simulink model "SVPWM"  (R2023b)
settings: Solver=FixedStepAuto  StartTime=0.0  StopTime=10.0  FixedStep=1e-4  RelTol=1e-3
undefined symbols (not defined in the file): curr_d_ki, curr_d_kp, curr_q_ki, curr_q_kp, CurrKi, CurrKp, Pn, Udc
libraries: slpidlib x4, mcbplantlib x1, autolibpmsmexterior x1
settings Model: DataDictionary=FOC.sldd  Creator=18575  LastModifiedBy=18575
settings OptimizationCC: DefaultParameterBehavior=Inlined  UseDivisionForNetSlopeComputation=on  GainParamInheritBuiltInType=on  UseFloatMulNetSlope=on  InlineInvariantSignals=on  PassReuseOutputArgsAs=Individual arguments  ZeroExternalMemoryAtStartup=off  ZeroInternalMemoryAtStartup=off  NoFixptDivByZeroProtection=on  EfficientFloat2IntCast=on  LifeSpan=1  OptimizeBlockOrder=speed  DifferentSizesBufferReuse=on  EfficientTunableParamExpr=on
settings DebuggingCC: ParameterTunabilityLossMsg=error
settings HardwareCC: ProdBitPerPointer=32  ProdBitPerSizeT=32  ProdBitPerPtrDiffT=32  ProdLargestAtomicInteger=Long  ProdLargestAtomicFloat=Double  ProdWordSize=32  ProdLongLongMode=on  ProdHWDeviceType=ARM Compatible->ARM Cortex-M
settings SFSimCC: MATLABDynamicMemAlloc=off
settings RTWCC: Description=Embedded Coder  SystemTargetFile=ert.tlc  TemplateMakefile=ert_default_tmf  GenerateReport=on  LaunchReport=on
settings CodeAppCC: ForceParamTrailComments=on  IgnoreCustomStorageClasses=off  OperatorAnnotations=on  SimulinkDataObjDesc=on  SFDataObjDesc=on  CustomSymbolStrGlobalVar=rt$N$M  CustomSymbolStrType=$N$M  CustomSymbolStrFcn=$N$M$F  CustomSymbolStrMacro=$N$M  InsertBlockDesc=on
settings ERTTargetCC: TargetLangStandard=C99 (ISO)  CodeReplacementLibrary=ARM Cortex-M  GenerateSampleERTMain=on  IncludeMdlTerminateFcn=off  CombineSignalStateStructs=on  SuppressErrorStatus=on  SupportAbsoluteTime=off  SupportNonFinite=off  SupportComplex=off  InlinedParameterPlacement=NonHierarchical  ERTCustomFileTemplate=example_file_process.tlc  ERTFilePackagingFormat=CompactWithDataFile

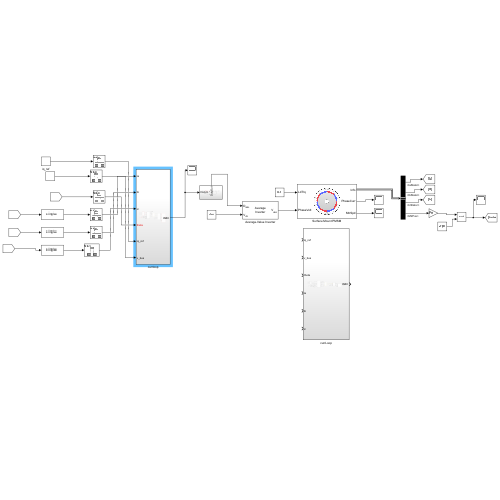
[thumbnail: Simulink's stored preview of the top-level diagram]
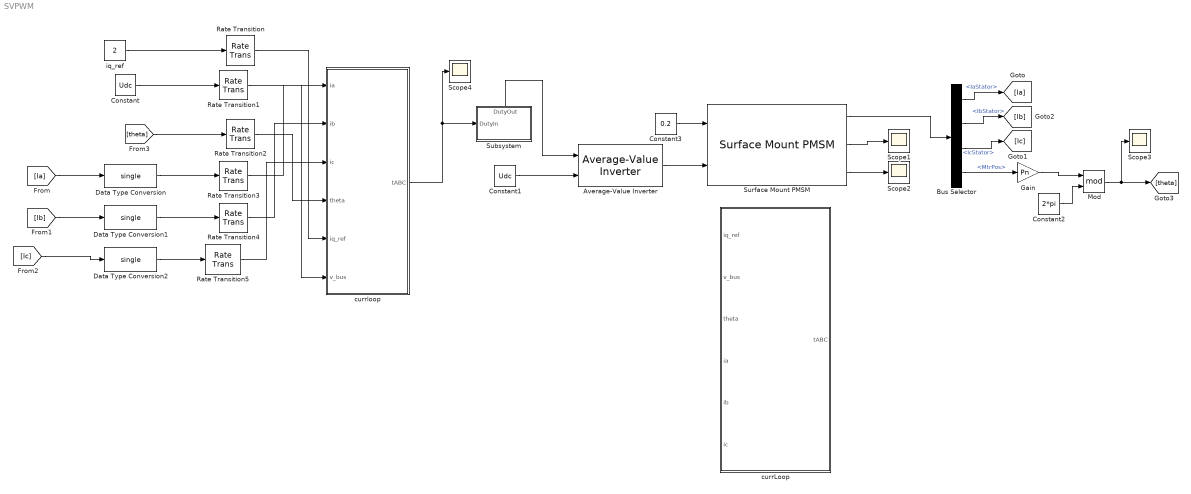
== system SVPWM ==
  Average-Value Inverter : mcbplantlib/Average-Value Inverter
      settings: LibrarySourceBlock=mcblib/Electrical Systems/Inverters/Average-Value Inverter
  Bus Selector : BusSelector  OutputSignals=IaStator,IbStator,IcStator,MtrPos
  Constant : Constant  Value=Udc
  Constant1 : Constant  Value=Udc
  Constant2 : Constant  Value=2*pi
  Constant3 : Constant  Value=0.2
  Data Type Conversion : DataTypeConversion  OutDataTypeStr=single  SaturateOnIntegerOverflow=off  RndMeth=Floor
  Data Type Conversion1 : DataTypeConversion  OutDataTypeStr=single  SaturateOnIntegerOverflow=off  RndMeth=Floor
  Data Type Conversion2 : DataTypeConversion  OutDataTypeStr=single  SaturateOnIntegerOverflow=off  RndMeth=Floor
  Gain : Gain  Gain=Pn
  Mod : Math  Operator=mod
  Rate Transition{,1..5} (6 alike) : RateTransition
  Scope{1..4} (4 alike) : Scope
  Subsystem : Subsystem
      settings: PortSchema="{\"entries\":[{\"content\":{\"sides\":[{\"content\":{\"connectorIds\":[\"In1\"]},\"type\":\"ConnectorPlacement.EquallySpacedRectSide\",\"uuid\":\"8ccc51de-fa2a-4900-80a3-4cdf9aa76f01\"},{\"content\":{\"side\":\"RIGHT\"},\"type\":\"ConnectorPlacement.EquallySpacedRectSide\",\"uuid\":\"32c06e0d-3f1d-4948-af96-e310e54308a0\"},{\"content\":{\"connectorIds\":[\"Out1\"],\"side\":\"TOP\"},\"type\":\"ConnectorPlacement.EquallySpacedRectSide\",\"uuid\":\"a9066067-2c54-42a8-b4d7-fb86ac71b860\"}]},\"type\":\"ConnectorPlacement.EquallySpacedConnector\",\"uuid\":\"e4576975-acad-4e16-822f-2c2e7f23d7a7\"}],\"packageUris\":[\"http://schema.mathworks.com/mf0/Connector/R2020b\"],\"version\":\"1.0\"}"
  Surface Mount PMSM : autolibpmsmexterior/Surface Mount PMSM  port_config=Torque  sim_type=Discrete  Ts=1e-4  FilePath=E:\Sandbox\Bauto\Work\surfacepmsm_motordata.m  P=Pn  Rs=Rs  Ldq_=L  KConstText=Permanent flux linkage constant (lambda_pm):  lambda_pm=flux  Ke=159.9771  Kt=1.323  mechanical=[75e-6, 8e-5, 0]  idq0=[0 0]  theta_init=0  omega_init=0  KConst=flux  lambda_pm_calc=flux  RefBlkName='autolibpmsmexterior/Surface Mount PMSM'  aMode=1  Ldq="[0.0003752   0.0003752]"
      settings: LibrarySourceBlock=autolibemachines/Surface Mount PMSM
  currLoop : Subsystem
  currloop : Subsystem
  iq_ref : Constant  Value=2  OutDataTypeStr=single
  wires:
  Average-Value Inverter/1 -> Surface Mount PMSM/2
  Surface Mount PMSM/3 -> Scope2/1
  Surface Mount PMSM/2 -> Scope1/1
  Surface Mount PMSM/1 -> Bus Selector/1
  iq_ref/1 -> Rate Transition/1
  Constant/1 -> Rate Transition1/1
  [theta] -> Rate Transition2/1
  currloop/1(tABC) -> Scope4/1, Subsystem/1(DutyIn)
  Subsystem/1(DutyOut) -> Average-Value Inverter/1
  [Ia] -> Data Type Conversion/1
  [Ic] -> Data Type Conversion2/1
  [Ib] -> Data Type Conversion1/1
  Data Type Conversion/1 -> Rate Transition3/1
  Data Type Conversion1/1 -> Rate Transition4/1
  Data Type Conversion2/1 -> Rate Transition5/1
  Rate Transition/1 -> currloop/5(iq_ref)
  Rate Transition1/1 -> currloop/6(v_bus)
  Rate Transition2/1 -> currloop/4(theta)
  Rate Transition3/1 -> currloop/1(ia)
  Rate Transition4/1 -> currloop/2(ib)
  Rate Transition5/1 -> currloop/3(ic)
  Bus Selector/1 -> [Ia]  "<IaStator>"
  Bus Selector/2 -> [Ib]  "<IbStator>"
  Bus Selector/3 -> [Ic]  "<IcStator>"
  Bus Selector/4 -> Gain/1  "<MtrPos>"
  Constant1/1 -> Average-Value Inverter/2
  Gain/1 -> Mod/1
  Constant2/1 -> Mod/2
  Mod/1 -> Scope3/1, [theta]
  Constant3/1 -> Surface Mount PMSM/1

== system SVPWM/Subsystem ==
  DutyIn : Inport
  Constant : Constant  Value=0.5  SampleTime=-1
  Gain : Gain  Gain=1/8000  ParamDataTypeStr=single
  Gain1 : Gain  Gain=-1
  Sum : Sum  Inputs=|+-
  Sum1 : Sum  Inputs=|++
  DutyOut : Outport
  wires:
  Sum/1 -> Gain1/1
  Constant/1 -> Sum1/2, Sum/2
  DutyIn/1 -> Gain/1
  Gain1/1 -> Sum1/1
  Sum1/1 -> DutyOut/1
  Gain/1 -> Sum/1

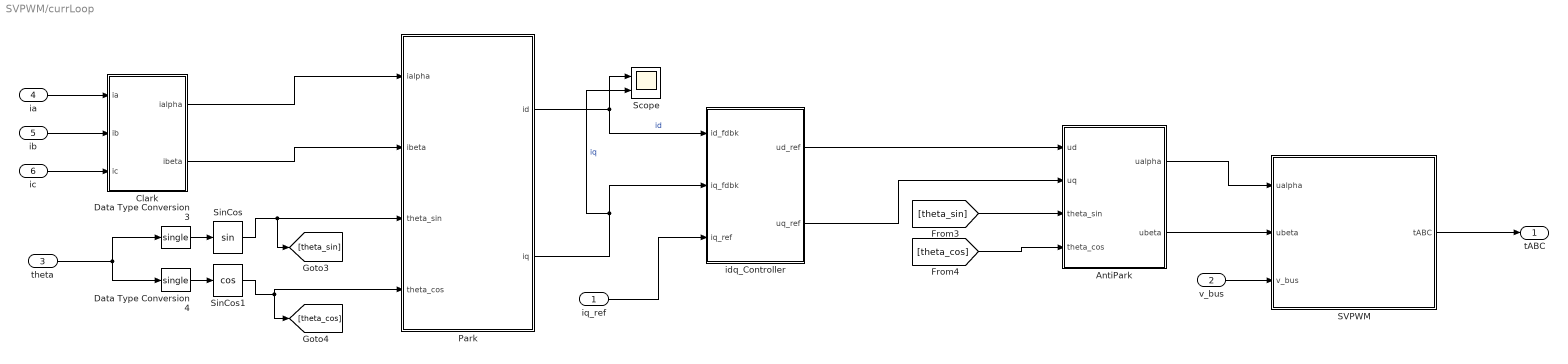
== system SVPWM/currLoop ==
  iq_ref : Inport
  v_bus : Inport  Port=2
  theta : Inport  Port=3
  ia : Inport  Port=4
  ib : Inport  Port=5
  ic : Inport  Port=6
  AntiPark : Subsystem
  Clark : Subsystem
  Data Type Conversion3 : DataTypeConversion  OutDataTypeStr=single  SaturateOnIntegerOverflow=off  RndMeth=Floor
  Data Type Conversion4 : DataTypeConversion  OutDataTypeStr=single  SaturateOnIntegerOverflow=off  RndMeth=Floor
  Park : Subsystem
  SVPWM : Subsystem
  Scope : Scope  NumInputPorts=2
  SinCos : Trigonometry
  SinCos1 : Trigonometry  Operator=cos
  idq_Controller : Subsystem
  tABC : Outport
  wires:
  v_bus/1 -> SVPWM/3(v_bus)
  Park/1(id) -> idq_Controller/1(id_fdbk), Scope/1  "id"
  SVPWM/1(tABC) -> tABC/1
  [theta_sin] -> AntiPark/3(theta_sin)
  SinCos/1 -> Park/3(theta_sin), [theta_sin]
  theta/1 -> Data Type Conversion4/1, Data Type Conversion3/1
  [theta_cos] -> AntiPark/4(theta_cos)
  idq_Controller/1(ud_ref) -> AntiPark/1(ud)
  SinCos1/1 -> Park/4(theta_cos), [theta_cos]
  AntiPark/2(ubeta) -> SVPWM/2(ubeta)
  AntiPark/1(ualpha) -> SVPWM/1(ualpha)
  idq_Controller/2(uq_ref) -> AntiPark/2(uq)
  Park/2(iq) -> idq_Controller/2(iq_fdbk), Scope/2  "iq"
  Clark/2(ibeta) -> Park/2(ibeta)
  iq_ref/1 -> idq_Controller/3(iq_ref)
  Clark/1(ialpha) -> Park/1(ialpha)
  Data Type Conversion4/1 -> SinCos1/1
  Data Type Conversion3/1 -> SinCos/1
  ia/1 -> Clark/1(ia)
  ib/1 -> Clark/2(ib)
  ic/1 -> Clark/3(ic)

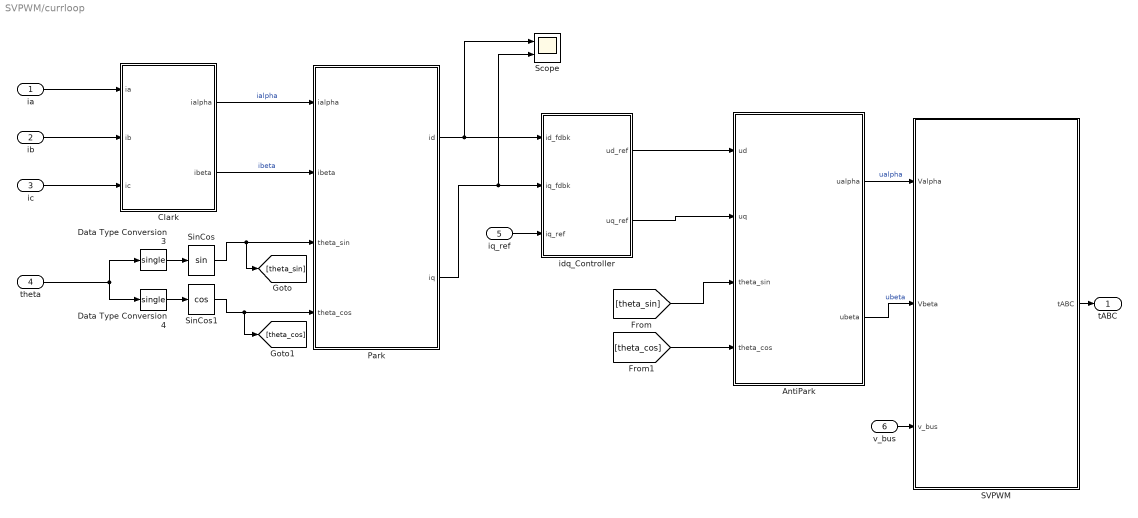
== system SVPWM/currloop ==
  ia : Inport
  ib : Inport  Port=2
  ic : Inport  Port=3
  theta : Inport  Port=4
  iq_ref : Inport  Port=5
  v_bus : Inport  Port=6
  AntiPark : Subsystem
  Clark : Subsystem
  Data Type Conversion3 : DataTypeConversion  OutDataTypeStr=single  SaturateOnIntegerOverflow=off  RndMeth=Floor
  Data Type Conversion4 : DataTypeConversion  OutDataTypeStr=single  SaturateOnIntegerOverflow=off  RndMeth=Floor
  Park : Subsystem
  SVPWM : Subsystem  TreatAsAtomicUnit=on
  Scope : Scope  NumInputPorts=2
  SinCos : Trigonometry
  SinCos1 : Trigonometry  Operator=cos
  idq_Controller : Subsystem
  tABC : Outport
  wires:
  Data Type Conversion4/1 -> SinCos1/1
  Data Type Conversion3/1 -> SinCos/1
  AntiPark/2(ubeta) -> SVPWM/2(Vbeta)  "ubeta"
  AntiPark/1(ualpha) -> SVPWM/1(Valpha)  "ualpha"
  [theta_cos] -> AntiPark/4(theta_cos)
  [theta_sin] -> AntiPark/3(theta_sin)
  SinCos/1 -> Park/3(theta_sin), [theta_sin]
  theta/1 -> Data Type Conversion3/1, Data Type Conversion4/1
  SinCos1/1 -> Park/4(theta_cos), [theta_cos]
  v_bus/1 -> SVPWM/3(v_bus)
  SVPWM/1(tABC) -> tABC/1
  ib/1 -> Clark/2(ib)
  ia/1 -> Clark/1(ia)
  ic/1 -> Clark/3(ic)
  Clark/1(ialpha) -> Park/1(ialpha)  "ialpha"
  Clark/2(ibeta) -> Park/2(ibeta)  "ibeta"
  idq_Controller/1(ud_ref) -> AntiPark/1(ud)
  idq_Controller/2(uq_ref) -> AntiPark/2(uq)
  Park/1(id) -> Scope/1, idq_Controller/1(id_fdbk)
  Park/2(iq) -> Scope/2, idq_Controller/2(iq_fdbk)
  iq_ref/1 -> idq_Controller/3(iq_ref)

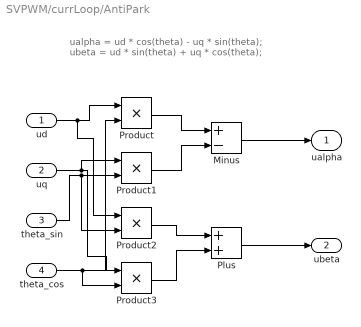
== system SVPWM/currLoop/AntiPark ==
  note: ualpha = ud * cos(theta) - uq * sin(theta);
      | ubeta = ud * sin(theta) + uq * cos(theta);
  ud : Inport
  uq : Inport  Port=2
  theta_sin : Inport  Port=3
  theta_cos : Inport  Port=4
  Minus : Sum  Inputs=+-
  Plus : Sum
  Product{,1..3} (4 alike) : Product
  ualpha : Outport
  ubeta : Outport  Port=2
  wires:
  ud/1 -> Product2/1, Product/1
  theta_cos/1 -> Product3/2, Product/2
  Product/1 -> Minus/1
  uq/1 -> Product3/1, Product1/1
  theta_sin/1 -> Product2/2, Product1/2
  Product1/1 -> Minus/2
  Minus/1 -> ualpha/1
  Product2/1 -> Plus/1
  Product3/1 -> Plus/2
  Plus/1 -> ubeta/1

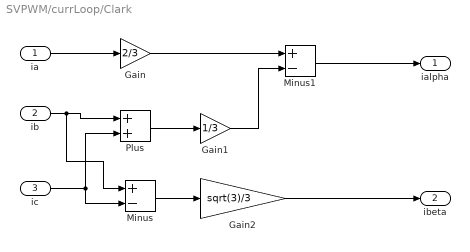
== system SVPWM/currLoop/Clark ==
  ia : Inport  OutDataTypeStr=single
  ib : Inport  Port=2  OutDataTypeStr=single
  ic : Inport  Port=3  OutDataTypeStr=single
  Gain : Gain  Gain=2/3
  Gain1 : Gain  Gain=1/3
  Gain2 : Gain  Gain=sqrt(3)/3
  Minus : Sum  Inputs=+-
  Minus1 : Sum  Inputs=+-
  Plus : Sum
  ialpha : Outport
  ibeta : Outport  Port=2
  wires:
  Gain/1 -> Minus1/1
  Plus/1 -> Gain1/1
  ic/1 -> Minus/2, Plus/2
  Gain1/1 -> Minus1/2
  Gain2/1 -> ibeta/1
  Minus1/1 -> ialpha/1
  ia/1 -> Gain/1
  Minus/1 -> Gain2/1
  ib/1 -> Minus/1, Plus/1

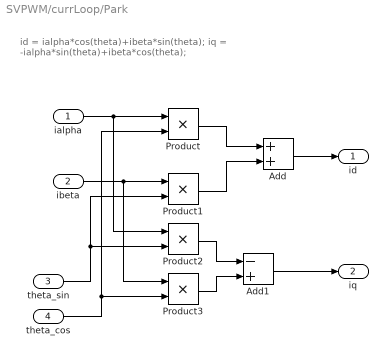
== system SVPWM/currLoop/Park ==
  note: id = ialpha*cos(theta)+ibeta*sin(theta);
      | iq = -ialpha*sin(theta)+ibeta*cos(theta);
  ialpha : Inport  OutDataTypeStr=single
  ibeta : Inport  Port=2  OutDataTypeStr=single
  theta_sin : Inport  Port=3  OutDataTypeStr=single
  theta_cos : Inport  Port=4  OutDataTypeStr=single
  Add : Sum  OutDataTypeStr=single  AccumDataTypeStr=single
  Add1 : Sum  Inputs=-+  OutDataTypeStr=single  AccumDataTypeStr=single
  Product{,1..3} (4 alike) : Product  OutDataTypeStr=single
  id : Outport  OutDataTypeStr=single
  iq : Outport  Port=2  OutDataTypeStr=single
  wires:
  theta_sin/1 -> Product2/2, Product1/2
  Product/1 -> Add/1
  Product2/1 -> Add1/1
  ialpha/1 -> Product2/1, Product/1
  Product3/1 -> Add1/2
  Add/1 -> id/1
  Add1/1 -> iq/1
  Product1/1 -> Add/2
  ibeta/1 -> Product3/1, Product1/1
  theta_cos/1 -> Product3/2, Product/2

== system SVPWM/currLoop/SVPWM ==
  ualpha : Inport
  ubeta : Inport  Port=2
  v_bus : Inport  Port=3
  AntiClark : Subsystem
  Divide : Product  Inputs=*/
  Mux : Mux  Inputs=3
  PWM_halfPeriod : Gain  Gain=8000
  Sum : Sum  Inputs=++|
  center : Subsystem
  tABC : Outport
  wires:
  AntiClark/1(Ua) -> Mux/1
  AntiClark/2(Ub) -> Mux/2
  AntiClark/3(Uc) -> Mux/3
  Mux/1 -> Sum/2, center/1(Uabc)
  center/1(Ucenter) -> Sum/1
  v_bus/1 -> Divide/2, center/2(v_bus)
  ualpha/1 -> AntiClark/1(ualpha)
  ubeta/1 -> AntiClark/2(ubeta)
  Sum/1 -> Divide/1
  Divide/1 -> PWM_halfPeriod/1
  PWM_halfPeriod/1 -> tABC/1

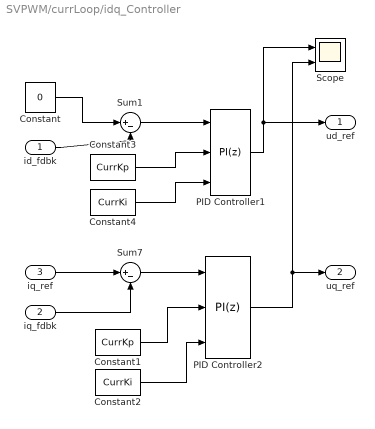
== system SVPWM/currLoop/idq_Controller ==
  id_fdbk : Inport  OutDataTypeStr=single
  iq_fdbk : Inport  Port=2  OutDataTypeStr=single
  iq_ref : Inport  Port=3  OutDataTypeStr=single
  Constant : Constant  Value=0  OutDataTypeStr=single
  Constant1 : Constant  Value=CurrKp  OutDataTypeStr=single
  Constant2 : Constant  Value=CurrKi  OutDataTypeStr=single
  Constant3 : Constant  Value=CurrKp  OutDataTypeStr=single
  Constant4 : Constant  Value=CurrKi  OutDataTypeStr=single
  PID Controller1 : slpidlib/PID Controller  Controller=PI  Form=Parallel  TimeDomain=Discrete-time  UseExternalTs=off  SampleTime=-1  IntegratorMethod=Forward Euler  FilterMethod=Forward Euler  ControllerParametersSource=external  P=curr_d_kp  I=curr_d_ki  UseKiTs=off  D=0  N=100  UseFilter=on  TunerSelectOption=Transfer Function Based (PID Tuner App)  InitialConditionSource=internal  InitialConditionForIntegrator=0  InitialConditionForFilter=0  DifferentiatorICPrevScaledInput=0  ExternalReset=none  TrackingMode=off  Kt=1  LimitOutput=on  SatLimitsSource=internal  UpperSaturationLimit=24*0.9/sqrt(3)  LowerSaturationLimit=-24*0.9/sqrt(3)  LinearizeAsGain=on  AntiWindupMode=clamping  Kb=1  LimitIntegrator=off  UpperIntegratorSaturationLimit=inf  LowerIntegratorSaturationLimit=-inf  PGainOutDataTypeStr=single  PProdOutDataTypeStr=single  POutMin=[]  POutMax=[]  IGainOutDataTypeStr=int16  IProdOutDataTypeStr=int16  IOutMin=[]  IOutMax=[]  DOutMin=[]  DOutMax=[]  NOutMin=[]  NOutMax=[]  SumOutDataTypeStr=single  SumOutMin=[]  SumOutMax=[]  SaturationOutDataTypeStr=single  SaturationOutMin=[]  SaturationOutMax=[]  PParamMin=[]  PParamMax=[]  IParamMin=[]  IParamMax=[]  DParamMin=[]  DParamMax=[]  NParamMin=[]  NParamMax=[]  KbParamMin=[]  KbParamMax=[]  KtParamMin=[]  KtParamMax=[]  KbOutMin=[]  KbOutMax=[]  KtOutMin=[]  KtOutMax=[]  IntegratorOutMin=[]  IntegratorOutMax=[]  FilterOutMin=[]  FilterOutMax=[]  SumI1OutMin=[]  SumI1OutMax=[]  SumI2OutMin=[]  SumI2OutMax=[]  SumI3OutMin=[]  SumI3OutMax=[]  SumI4OutMin=[]  SumI4OutMax=[]  SumDOutMin=[]  SumDOutMax=[]  DifferentiatorOutMin=[]  DifferentiatorOutMax=[]  FilterDiffOutCoefMin=[]  FilterDiffOutCoefMax=[]  ReciprocalOutMin=[]  ReciprocalOutMax=[]  SumDenOutMin=[]  SumDenOutMax=[]  SumNumOutMin=[]  SumNumOutMax=[]  DivideOutMin=[]  DivideOutMax=[]  UdiffTsProdOutMin=[]  UdiffTsProdOutMax=[]  NTsProdOutMin=[]  NTsProdOutMax=[]  UintegralTsProdOutMin=[]  UintegralTsProdOutMax=[]  UngainTsProdOutMin=[]  UngainTsProdOutMax=[]  ClampingZeroOutDataTypeStr=Inherit: Inherit via back propagation  ClampingZeroOutMin=[]  ClampingZeroOutMax=[]  FilterDenConstantOutDataTypeStr=Inherit: Inherit via back propagation  FilterDenConstantOutMin=[]  FilterDenConstantOutMax=[]  PCopyOutDataTypeStr=Inherit: Inherit via back propagation  PCopyOutMin=[]  PCopyOutMax=[]  NCopyOutDataTypeStr=Inherit: Inherit via back propagation  NCopyOutMin=[]  NCopyOutMax=[]  IntegratorContinuousStateAttributes=''  IntegratorStateMustResolveToSignalObject=off  IntegratorRTWStateStorageClass=Auto  FilterContinuousStateAttributes=''  FilterStateMustResolveToSignalObject=off  FilterRTWStateStorageClass=Auto  ParallelPVariant=ExternalParameters  IdealPVariant=Disabled  IVariant=ExternalParameters  DVariant=Disabled  IntegratorVariant=Discrete  SatVariant=Enabled  AWVariant=DiscClampingParallel  PCopyVariant=Disabled  TRVariant=Disabled  FdbkBlocksVariant=Forward  IdealPFdbkVariant=Disabled  SatFdbkVariant=Disabled  DerivativeFilterVariant=Disabled  NVariant=Disabled  NCopyVariant=Disabled_SignalSpec  FilterICVariant=Disabled  IntegratorICVariant=InternalICs  ExternalResetVariant=Disabled  TRSumVariant=Passthrough  SumFdbkVariant=Disabled  SumVariant=Sum_PI  TsampFilterVariant=InternalTs  TsampNgainVariant=Passthrough  TsampIntegralVariant=Disabled_SignalSpec  ExternalSaturationOutDataTypeStr=Inherit: Same as second input
  PID Controller2 : slpidlib/PID Controller  Controller=PI  Form=Parallel  TimeDomain=Discrete-time  UseExternalTs=off  SampleTime=-1  IntegratorMethod=Forward Euler  FilterMethod=Forward Euler  ControllerParametersSource=external  P=curr_q_kp  I=curr_q_ki  UseKiTs=off  D=0  N=100  UseFilter=on  TunerSelectOption=Transfer Function Based (PID Tuner App)  InitialConditionSource=internal  InitialConditionForIntegrator=0  InitialConditionForFilter=0  DifferentiatorICPrevScaledInput=0  ExternalReset=none  TrackingMode=off  Kt=1  LimitOutput=on  SatLimitsSource=internal  UpperSaturationLimit=24*0.9/sqrt(3)  LowerSaturationLimit=-24*0.9/sqrt(3)  LinearizeAsGain=on  AntiWindupMode=clamping  Kb=1  LimitIntegrator=off  UpperIntegratorSaturationLimit=inf  LowerIntegratorSaturationLimit=-inf  PGainOutDataTypeStr=single  PProdOutDataTypeStr=single  POutMin=[]  POutMax=[]  IGainOutDataTypeStr=single  IProdOutDataTypeStr=single  IOutMin=[]  IOutMax=[]  DOutMin=[]  DOutMax=[]  NOutMin=[]  NOutMax=[]  SumOutDataTypeStr=single  SumOutMin=[]  SumOutMax=[]  SaturationOutDataTypeStr=single  SaturationOutMin=[]  SaturationOutMax=[]  PParamMin=[]  PParamMax=[]  IParamMin=[]  IParamMax=[]  DParamMin=[]  DParamMax=[]  NParamMin=[]  NParamMax=[]  KbParamMin=[]  KbParamMax=[]  KtParamMin=[]  KtParamMax=[]  KbOutMin=[]  KbOutMax=[]  KtOutMin=[]  KtOutMax=[]  IntegratorOutMin=[]  IntegratorOutMax=[]  FilterOutMin=[]  FilterOutMax=[]  SumI1OutMin=[]  SumI1OutMax=[]  SumI2OutMin=[]  SumI2OutMax=[]  SumI3OutMin=[]  SumI3OutMax=[]  SumI4OutMin=[]  SumI4OutMax=[]  SumDOutMin=[]  SumDOutMax=[]  DifferentiatorOutMin=[]  DifferentiatorOutMax=[]  FilterDiffOutCoefMin=[]  FilterDiffOutCoefMax=[]  ReciprocalOutMin=[]  ReciprocalOutMax=[]  SumDenOutMin=[]  SumDenOutMax=[]  SumNumOutMin=[]  SumNumOutMax=[]  DivideOutMin=[]  DivideOutMax=[]  UdiffTsProdOutMin=[]  UdiffTsProdOutMax=[]  NTsProdOutMin=[]  NTsProdOutMax=[]  UintegralTsProdOutMin=[]  UintegralTsProdOutMax=[]  UngainTsProdOutMin=[]  UngainTsProdOutMax=[]  ClampingZeroOutDataTypeStr=Inherit: Inherit via back propagation  ClampingZeroOutMin=[]  ClampingZeroOutMax=[]  FilterDenConstantOutDataTypeStr=Inherit: Inherit via back propagation  FilterDenConstantOutMin=[]  FilterDenConstantOutMax=[]  PCopyOutDataTypeStr=Inherit: Inherit via back propagation  PCopyOutMin=[]  PCopyOutMax=[]  NCopyOutDataTypeStr=Inherit: Inherit via back propagation  NCopyOutMin=[]  NCopyOutMax=[]  IntegratorContinuousStateAttributes=''  IntegratorStateMustResolveToSignalObject=off  IntegratorRTWStateStorageClass=Auto  FilterContinuousStateAttributes=''  FilterStateMustResolveToSignalObject=off  FilterRTWStateStorageClass=Auto  ParallelPVariant=ExternalParameters  IdealPVariant=Disabled  IVariant=ExternalParameters  DVariant=Disabled  IntegratorVariant=Discrete  SatVariant=Enabled  AWVariant=DiscClampingParallel  PCopyVariant=Disabled  TRVariant=Disabled  FdbkBlocksVariant=Forward  IdealPFdbkVariant=Disabled  SatFdbkVariant=Disabled  DerivativeFilterVariant=Disabled  NVariant=Disabled  NCopyVariant=Disabled_SignalSpec  FilterICVariant=Disabled  IntegratorICVariant=InternalICs  ExternalResetVariant=Disabled  TRSumVariant=Passthrough  SumFdbkVariant=Disabled  SumVariant=Sum_PI  TsampFilterVariant=InternalTs  TsampNgainVariant=Passthrough  TsampIntegralVariant=Disabled_SignalSpec  ExternalSaturationOutDataTypeStr=Inherit: Same as second input
  Scope : Scope  NumInputPorts=2
  Sum1 : Sum  Inputs=|+-  OutDataTypeStr=single  AccumDataTypeStr=single
  Sum7 : Sum  Inputs=|+-  OutDataTypeStr=single  AccumDataTypeStr=single
  ud_ref : Outport  OutDataTypeStr=single
  uq_ref : Outport  Port=2  OutDataTypeStr=single
  wires:
  id_fdbk/1 -> Sum1/2
  Constant/1 -> Sum1/1
  iq_fdbk/1 -> Sum7/2
  Sum1/1 -> PID Controller1/1
  Sum7/1 -> PID Controller2/1
  PID Controller1/1 -> Scope/1, ud_ref/1
  PID Controller2/1 -> Scope/2, uq_ref/1
  iq_ref/1 -> Sum7/1
  Constant3/1 -> PID Controller1/2
  Constant4/1 -> PID Controller1/3
  Constant1/1 -> PID Controller2/2
  Constant2/1 -> PID Controller2/3

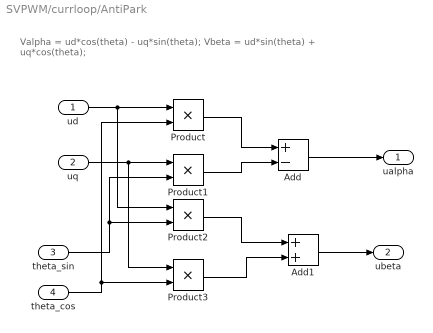
== system SVPWM/currloop/AntiPark ==
  note: Valpha = ud*cos(theta) - uq*sin(theta);
      | Vbeta = ud*sin(theta) + uq*cos(theta);
  ud : Inport
  uq : Inport  Port=2
  theta_sin : Inport  Port=3
  theta_cos : Inport  Port=4
  Add : Sum  Inputs=+-
  Add1 : Sum
  Product{,1..3} (4 alike) : Product
  ualpha : Outport  OutDataTypeStr=single
  ubeta : Outport  Port=2  OutDataTypeStr=single
  wires:
  Product2/1 -> Add1/1
  Product/1 -> Add/1
  Add/1 -> ualpha/1
  Product3/1 -> Add1/2
  ud/1 -> Product/1, Product2/1
  theta_sin/1 -> Product1/2, Product2/2
  theta_cos/1 -> Product3/2, Product/2
  uq/1 -> Product1/1, Product3/1
  Product1/1 -> Add/2
  Add1/1 -> ubeta/1

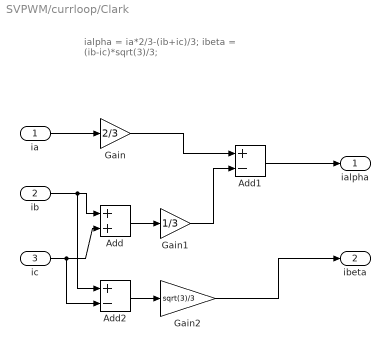
== system SVPWM/currloop/Clark ==
  note: ialpha = ia*2/3-(ib+ic)/3;
      | ibeta = (ib-ic)*sqrt(3)/3;
  ia : Inport  OutDataTypeStr=single
  ib : Inport  Port=2  OutDataTypeStr=single
  ic : Inport  Port=3  OutDataTypeStr=single
  Add : Sum  OutDataTypeStr=single  AccumDataTypeStr=single
  Add1 : Sum  Inputs=+-  OutDataTypeStr=single  AccumDataTypeStr=single
  Add2 : Sum  Inputs=+-  OutDataTypeStr=single  AccumDataTypeStr=single
  Gain : Gain  Gain=2/3  ParamDataTypeStr=single
  Gain1 : Gain  Gain=1/3  ParamDataTypeStr=single
  Gain2 : Gain  Gain=sqrt(3)/3  ParamDataTypeStr=single
  ialpha : Outport  OutDataTypeStr=single
  ibeta : Outport  Port=2  OutDataTypeStr=single
  wires:
  Add1/1 -> ialpha/1
  ia/1 -> Gain/1
  Gain2/1 -> ibeta/1
  ib/1 -> Add/1, Add2/1
  Gain/1 -> Add1/1
  Add2/1 -> Gain2/1
  Add/1 -> Gain1/1
  ic/1 -> Add/2, Add2/2
  Gain1/1 -> Add1/2

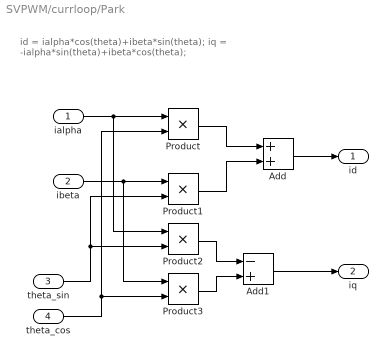
== system SVPWM/currloop/Park ==
  note: id = ialpha*cos(theta)+ibeta*sin(theta);
      | iq = -ialpha*sin(theta)+ibeta*cos(theta);
  ialpha : Inport  OutDataTypeStr=single
  ibeta : Inport  Port=2  OutDataTypeStr=single
  theta_sin : Inport  Port=3  OutDataTypeStr=single
  theta_cos : Inport  Port=4  OutDataTypeStr=single
  Add : Sum  OutDataTypeStr=single  AccumDataTypeStr=single
  Add1 : Sum  Inputs=-+  OutDataTypeStr=single  AccumDataTypeStr=single
  Product{,1..3} (4 alike) : Product  OutDataTypeStr=single
  id : Outport  OutDataTypeStr=single
  iq : Outport  Port=2  OutDataTypeStr=single
  wires:
  theta_cos/1 -> Product/2, Product3/2
  ibeta/1 -> Product1/1, Product3/1
  Product1/1 -> Add/2
  Add1/1 -> iq/1
  Add/1 -> id/1
  Product3/1 -> Add1/2
  ialpha/1 -> Product/1, Product2/1
  Product2/1 -> Add1/1
  Product/1 -> Add/1
  theta_sin/1 -> Product1/2, Product2/2

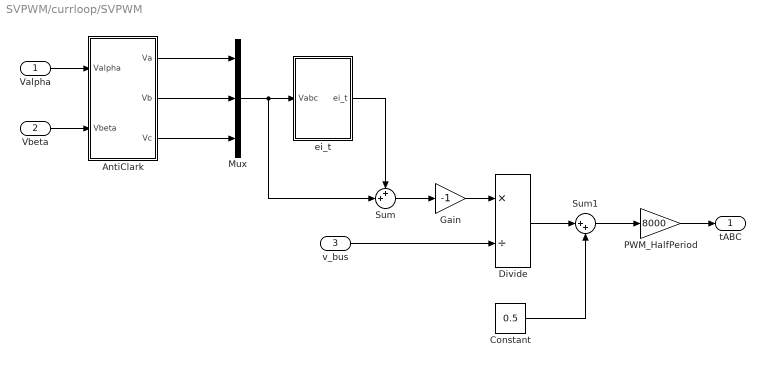
== system SVPWM/currloop/SVPWM ==
  Valpha : Inport  OutDataTypeStr=single
  Vbeta : Inport  Port=2  OutDataTypeStr=single
  v_bus : Inport  Port=3  OutDataTypeStr=single
  AntiClark : Subsystem
  Constant : Constant  Value=0.5  OutDataTypeStr=single
  Divide : Product  Inputs=*/  OutDataTypeStr=single
  Gain : Gain  Gain=-1  OutDataTypeStr=single
  Mux : Mux  Inputs=3
  PWM_HalfPeriod : Gain  Gain=8000  OutDataTypeStr=single
  Sum : Sum  Inputs=++|  OutDataTypeStr=single
  Sum1 : Sum  Inputs=|++  OutDataTypeStr=single
  ei_t : Subsystem
  tABC : Outport  OutDataTypeStr=single
  wires:
  Gain/1 -> Divide/1
  v_bus/1 -> Divide/2
  PWM_HalfPeriod/1 -> tABC/1
  Sum1/1 -> PWM_HalfPeriod/1
  Constant/1 -> Sum1/2
  Divide/1 -> Sum1/1
  Mux/1 -> ei_t/1(Vabc), Sum/2
  Sum/1 -> Gain/1
  AntiClark/3(Vc) -> Mux/3
  AntiClark/2(Vb) -> Mux/2
  AntiClark/1(Va) -> Mux/1
  ei_t/1(ei_t) -> Sum/1
  Vbeta/1 -> AntiClark/2(Vbeta)
  Valpha/1 -> AntiClark/1(Valpha)

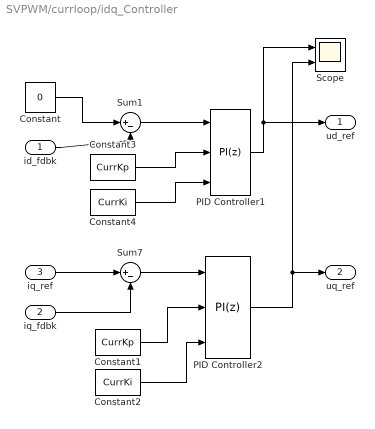
== system SVPWM/currloop/idq_Controller ==
  id_fdbk : Inport  OutDataTypeStr=single
  iq_fdbk : Inport  Port=2  OutDataTypeStr=single
  iq_ref : Inport  Port=3  OutDataTypeStr=single
  Constant : Constant  Value=0  OutDataTypeStr=single
  Constant1 : Constant  Value=CurrKp  OutDataTypeStr=single
  Constant2 : Constant  Value=CurrKi  OutDataTypeStr=single
  Constant3 : Constant  Value=CurrKp  OutDataTypeStr=single
  Constant4 : Constant  Value=CurrKi  OutDataTypeStr=single
  PID Controller1 : slpidlib/PID Controller  Controller=PI  Form=Parallel  TimeDomain=Discrete-time  UseExternalTs=off  SampleTime=-1  IntegratorMethod=Forward Euler  FilterMethod=Forward Euler  ControllerParametersSource=external  P=curr_d_kp  I=curr_d_ki  UseKiTs=off  D=0  N=100  UseFilter=on  TunerSelectOption=Transfer Function Based (PID Tuner App)  InitialConditionSource=internal  InitialConditionForIntegrator=0  InitialConditionForFilter=0  DifferentiatorICPrevScaledInput=0  ExternalReset=none  TrackingMode=off  Kt=1  LimitOutput=on  SatLimitsSource=internal  UpperSaturationLimit=24*0.9/sqrt(3)  LowerSaturationLimit=-24*0.9/sqrt(3)  LinearizeAsGain=on  AntiWindupMode=clamping  Kb=1  LimitIntegrator=off  UpperIntegratorSaturationLimit=inf  LowerIntegratorSaturationLimit=-inf  PGainOutDataTypeStr=single  PProdOutDataTypeStr=single  POutMin=[]  POutMax=[]  IGainOutDataTypeStr=int16  IProdOutDataTypeStr=int16  IOutMin=[]  IOutMax=[]  DOutMin=[]  DOutMax=[]  NOutMin=[]  NOutMax=[]  SumOutDataTypeStr=single  SumOutMin=[]  SumOutMax=[]  SaturationOutDataTypeStr=single  SaturationOutMin=[]  SaturationOutMax=[]  PParamMin=[]  PParamMax=[]  IParamMin=[]  IParamMax=[]  DParamMin=[]  DParamMax=[]  NParamMin=[]  NParamMax=[]  KbParamMin=[]  KbParamMax=[]  KtParamMin=[]  KtParamMax=[]  KbOutMin=[]  KbOutMax=[]  KtOutMin=[]  KtOutMax=[]  IntegratorOutMin=[]  IntegratorOutMax=[]  FilterOutMin=[]  FilterOutMax=[]  SumI1OutMin=[]  SumI1OutMax=[]  SumI2OutMin=[]  SumI2OutMax=[]  SumI3OutMin=[]  SumI3OutMax=[]  SumI4OutMin=[]  SumI4OutMax=[]  SumDOutMin=[]  SumDOutMax=[]  DifferentiatorOutMin=[]  DifferentiatorOutMax=[]  FilterDiffOutCoefMin=[]  FilterDiffOutCoefMax=[]  ReciprocalOutMin=[]  ReciprocalOutMax=[]  SumDenOutMin=[]  SumDenOutMax=[]  SumNumOutMin=[]  SumNumOutMax=[]  DivideOutMin=[]  DivideOutMax=[]  UdiffTsProdOutMin=[]  UdiffTsProdOutMax=[]  NTsProdOutMin=[]  NTsProdOutMax=[]  UintegralTsProdOutMin=[]  UintegralTsProdOutMax=[]  UngainTsProdOutMin=[]  UngainTsProdOutMax=[]  ClampingZeroOutDataTypeStr=Inherit: Inherit via back propagation  ClampingZeroOutMin=[]  ClampingZeroOutMax=[]  FilterDenConstantOutDataTypeStr=Inherit: Inherit via back propagation  FilterDenConstantOutMin=[]  FilterDenConstantOutMax=[]  PCopyOutDataTypeStr=Inherit: Inherit via back propagation  PCopyOutMin=[]  PCopyOutMax=[]  NCopyOutDataTypeStr=Inherit: Inherit via back propagation  NCopyOutMin=[]  NCopyOutMax=[]  IntegratorContinuousStateAttributes=''  IntegratorStateMustResolveToSignalObject=off  IntegratorRTWStateStorageClass=Auto  FilterContinuousStateAttributes=''  FilterStateMustResolveToSignalObject=off  FilterRTWStateStorageClass=Auto  ParallelPVariant=ExternalParameters  IdealPVariant=Disabled  IVariant=ExternalParameters  DVariant=Disabled  IntegratorVariant=Discrete  SatVariant=Enabled  AWVariant=DiscClampingParallel  PCopyVariant=Disabled  TRVariant=Disabled  FdbkBlocksVariant=Forward  IdealPFdbkVariant=Disabled  SatFdbkVariant=Disabled  DerivativeFilterVariant=Disabled  NVariant=Disabled  NCopyVariant=Disabled_SignalSpec  FilterICVariant=Disabled  IntegratorICVariant=InternalICs  ExternalResetVariant=Disabled  TRSumVariant=Passthrough  SumFdbkVariant=Disabled  SumVariant=Sum_PI  TsampFilterVariant=InternalTs  TsampNgainVariant=Passthrough  TsampIntegralVariant=Disabled_SignalSpec  ExternalSaturationOutDataTypeStr=Inherit: Same as second input
  PID Controller2 : slpidlib/PID Controller  Controller=PI  Form=Parallel  TimeDomain=Discrete-time  UseExternalTs=off  SampleTime=-1  IntegratorMethod=Forward Euler  FilterMethod=Forward Euler  ControllerParametersSource=external  P=curr_q_kp  I=curr_q_ki  UseKiTs=off  D=0  N=100  UseFilter=on  TunerSelectOption=Transfer Function Based (PID Tuner App)  InitialConditionSource=internal  InitialConditionForIntegrator=0  InitialConditionForFilter=0  DifferentiatorICPrevScaledInput=0  ExternalReset=none  TrackingMode=off  Kt=1  LimitOutput=on  SatLimitsSource=internal  UpperSaturationLimit=24*0.9/sqrt(3)  LowerSaturationLimit=-24*0.9/sqrt(3)  LinearizeAsGain=on  AntiWindupMode=clamping  Kb=1  LimitIntegrator=off  UpperIntegratorSaturationLimit=inf  LowerIntegratorSaturationLimit=-inf  PGainOutDataTypeStr=single  PProdOutDataTypeStr=single  POutMin=[]  POutMax=[]  IGainOutDataTypeStr=single  IProdOutDataTypeStr=single  IOutMin=[]  IOutMax=[]  DOutMin=[]  DOutMax=[]  NOutMin=[]  NOutMax=[]  SumOutDataTypeStr=single  SumOutMin=[]  SumOutMax=[]  SaturationOutDataTypeStr=single  SaturationOutMin=[]  SaturationOutMax=[]  PParamMin=[]  PParamMax=[]  IParamMin=[]  IParamMax=[]  DParamMin=[]  DParamMax=[]  NParamMin=[]  NParamMax=[]  KbParamMin=[]  KbParamMax=[]  KtParamMin=[]  KtParamMax=[]  KbOutMin=[]  KbOutMax=[]  KtOutMin=[]  KtOutMax=[]  IntegratorOutMin=[]  IntegratorOutMax=[]  FilterOutMin=[]  FilterOutMax=[]  SumI1OutMin=[]  SumI1OutMax=[]  SumI2OutMin=[]  SumI2OutMax=[]  SumI3OutMin=[]  SumI3OutMax=[]  SumI4OutMin=[]  SumI4OutMax=[]  SumDOutMin=[]  SumDOutMax=[]  DifferentiatorOutMin=[]  DifferentiatorOutMax=[]  FilterDiffOutCoefMin=[]  FilterDiffOutCoefMax=[]  ReciprocalOutMin=[]  ReciprocalOutMax=[]  SumDenOutMin=[]  SumDenOutMax=[]  SumNumOutMin=[]  SumNumOutMax=[]  DivideOutMin=[]  DivideOutMax=[]  UdiffTsProdOutMin=[]  UdiffTsProdOutMax=[]  NTsProdOutMin=[]  NTsProdOutMax=[]  UintegralTsProdOutMin=[]  UintegralTsProdOutMax=[]  UngainTsProdOutMin=[]  UngainTsProdOutMax=[]  ClampingZeroOutDataTypeStr=Inherit: Inherit via back propagation  ClampingZeroOutMin=[]  ClampingZeroOutMax=[]  FilterDenConstantOutDataTypeStr=Inherit: Inherit via back propagation  FilterDenConstantOutMin=[]  FilterDenConstantOutMax=[]  PCopyOutDataTypeStr=Inherit: Inherit via back propagation  PCopyOutMin=[]  PCopyOutMax=[]  NCopyOutDataTypeStr=Inherit: Inherit via back propagation  NCopyOutMin=[]  NCopyOutMax=[]  IntegratorContinuousStateAttributes=''  IntegratorStateMustResolveToSignalObject=off  IntegratorRTWStateStorageClass=Auto  FilterContinuousStateAttributes=''  FilterStateMustResolveToSignalObject=off  FilterRTWStateStorageClass=Auto  ParallelPVariant=ExternalParameters  IdealPVariant=Disabled  IVariant=ExternalParameters  DVariant=Disabled  IntegratorVariant=Discrete  SatVariant=Enabled  AWVariant=DiscClampingParallel  PCopyVariant=Disabled  TRVariant=Disabled  FdbkBlocksVariant=Forward  IdealPFdbkVariant=Disabled  SatFdbkVariant=Disabled  DerivativeFilterVariant=Disabled  NVariant=Disabled  NCopyVariant=Disabled_SignalSpec  FilterICVariant=Disabled  IntegratorICVariant=InternalICs  ExternalResetVariant=Disabled  TRSumVariant=Passthrough  SumFdbkVariant=Disabled  SumVariant=Sum_PI  TsampFilterVariant=InternalTs  TsampNgainVariant=Passthrough  TsampIntegralVariant=Disabled_SignalSpec  ExternalSaturationOutDataTypeStr=Inherit: Same as second input
  Scope : Scope  NumInputPorts=2
  Sum1 : Sum  Inputs=|+-  OutDataTypeStr=single  AccumDataTypeStr=single
  Sum7 : Sum  Inputs=|+-  OutDataTypeStr=single  AccumDataTypeStr=single
  ud_ref : Outport  OutDataTypeStr=single
  uq_ref : Outport  Port=2  OutDataTypeStr=single
  wires:
  id_fdbk/1 -> Sum1/2
  Constant/1 -> Sum1/1
  iq_fdbk/1 -> Sum7/2
  Sum1/1 -> PID Controller1/1
  Sum7/1 -> PID Controller2/1
  PID Controller1/1 -> Scope/1, ud_ref/1
  PID Controller2/1 -> Scope/2, uq_ref/1
  iq_ref/1 -> Sum7/1
  Constant3/1 -> PID Controller1/2
  Constant4/1 -> PID Controller1/3
  Constant1/1 -> PID Controller2/2
  Constant2/1 -> PID Controller2/3

== system SVPWM/currLoop/SVPWM/AntiClark ==
  note: Ua = ualpha;
      | Ub = ualpha * (-1/2) + ubeta *sqrt(3)/2;
      | Uc = ualpha * (-1/2) - ubeta * sqrt(3)/2;
  ualpha : Inport
  ubeta : Inport  Port=2
  Gain : Gain  Gain=-1/2
  Gain1 : Gain  Gain=sqrt(3)/2
  Sum : Sum  Inputs=|++
  Sum1 : Sum  Inputs=-+|
  Ua : Outport
  Ub : Outport  Port=2
  Uc : Outport  Port=3
  wires:
  ualpha/1 -> Gain/1, Ua/1
  ubeta/1 -> Gain1/1
  Gain/1 -> Sum1/2, Sum/1
  Gain1/1 -> Sum1/1, Sum/2
  Sum/1 -> Ub/1
  Sum1/1 -> Uc/1

== system SVPWM/currLoop/SVPWM/center ==
  note: U0 = -1/2(Umax + Umin);
      | Ucenter = v_bus / 2 + U0;
  Uabc : Inport
  v_bus : Inport  Port=2
  Demux : Demux  Outputs=3
  Gain : Gain  Gain=-1/2
  Gain1 : Gain  Gain=1/2
  Max : MinMax  Function=max  Inputs=3
  Min : MinMax  Inputs=3
  Sum : Sum  Inputs=|++
  Sum1 : Sum  Inputs=++|
  Ucenter : Outport
  wires:
  Uabc/1 -> Demux/1
  Demux/1 -> Max/1, Min/1
  Demux/2 -> Min/2, Max/2
  Demux/3 -> Min/3, Max/3
  Min/1 -> Sum/1
  Max/1 -> Sum/2
  Sum/1 -> Gain/1
  Gain/1 -> Sum1/1
  v_bus/1 -> Gain1/1
  Gain1/1 -> Sum1/2
  Sum1/1 -> Ucenter/1

== system SVPWM/currloop/SVPWM/AntiClark ==
  note: Va = Valpha;
      | Vb = Valpha*(-1/2)+Vbeta*sqrt(3)/3
      | Vc = Valpha*(-1/2)-Vbeta*sqrt(3)/3
  Valpha : Inport  OutDataTypeStr=single
  Vbeta : Inport  Port=2  OutDataTypeStr=single
  Gain : Gain  Gain=-1/2  OutDataTypeStr=single
  Gain1 : Gain  Gain=sqrt(3)/2  OutDataTypeStr=single
  Sum : Sum  Inputs=|++  OutDataTypeStr=single
  Sum1 : Sum  Inputs=-+|  OutDataTypeStr=single
  Va : Outport  OutDataTypeStr=single
  Vb : Outport  Port=2  OutDataTypeStr=single
  Vc : Outport  Port=3  OutDataTypeStr=single
  wires:
  Sum1/1 -> Vc/1
  Gain1/1 -> Sum1/1, Sum/2
  Sum/1 -> Vb/1
  Gain/1 -> Sum/1, Sum1/2
  Vbeta/1 -> Gain1/1
  Valpha/1 -> Va/1, Gain/1

== system SVPWM/currloop/SVPWM/ei_t ==
  note: V0 = -1/2(Vmax+Vmin)
  Vabc : Inport  OutDataTypeStr=single
  Demux : Demux  Outputs=3
  Gain : Gain  Gain=-1/2  OutDataTypeStr=single
  Min : MinMax  Inputs=3  OutDataTypeStr=single
  Min1 : MinMax  Function=max  Inputs=3  OutDataTypeStr=single
  Sum : Sum  Inputs=|++  OutDataTypeStr=single
  ei_t : Outport  OutDataTypeStr=single
  wires:
  Demux/3 -> Min/3, Min1/3
  Demux/2 -> Min1/2, Min/2
  Demux/1 -> Min/1, Min1/1
  Vabc/1 -> Demux/1
  Gain/1 -> ei_t/1
  Min1/1 -> Sum/2
  Sum/1 -> Gain/1
  Min/1 -> Sum/1
